simulink model "TSR_EuroNCAP_MSA_ISA_cs"  (R2014b)
settings: Solver=ode5  SolverMode=SingleTasking  StartTime=0.0  StopTime=inf  FixedStep=1/100  RelTol=1e-3
PreLoadFcn:
  | mbxruntime.callbacks.PreLoadFcn(bdroot);
  | check_NUTS_defined;
  | 
  | assignin('base',['model_closed_' bdroot],false);
  | 
  | addpath('../includes_TSR/includes_TSR');
  | 
  | 
  | switch version('-release')
  | case {'2010a', '2010b', '2011a'}
  | addpath('../includes_TSR/ML2010b');
  | otherwise
  | addpath('../includes_TSR/ML2011b');
  | end
PostLoadFcn:
  | mbxruntime.callbacks.PostLoadFcn(bdroot);
InitFcn:
  | mbxruntime.callbacks.InitFcn(bdroot);
StartFcn:
  | mbxruntime.callbacks.StartFcn(bdroot);
StopFcn:
  | mbxruntime.callbacks.StopFcn(bdroot);
model workspace: external: MAT-File .\TSR_EuroNCAP_MSA_ISA_cs_hws.mat (data not in the file)
undefined symbols (not defined in the file or in its folder): InitImageOutputDir, OrientationPitch, OrientationRoll, PositionX, PositionY, PositionZ, warningInitialVelocity, x0
undefined symbols (not defined in the file): SteeringColumn, SteeringWheel, TSR_EuroNCAP_MSA_ISA_cs_0104b7ba9617df32, TSR_EuroNCAP_MSA_ISA_cs_06e8a6c26bfd692b, TSR_EuroNCAP_MSA_ISA_cs_604176ef024b1671, TSR_EuroNCAP_MSA_ISA_cs_9eda5ebf0debb72b, TSR_EuroNCAP_MSA_ISA_cs_aae36e5db6336e11, TSR_EuroNCAP_MSA_ISA_cs_Audi_A8_1_Dynamics_Simple_initialPitch, TSR_EuroNCAP_MSA_ISA_cs_Audi_A8_1_Dynamics_Simple_initialRoll, TSR_EuroNCAP_MSA_ISA_cs_Audi_A8_1_Dynamics_Simple_initialX, TSR_EuroNCAP_MSA_ISA_cs_Audi_A8_1_Dynamics_Simple_initialY, TSR_EuroNCAP_MSA_ISA_cs_Audi_A8_1_Dynamics_Simple_initialYaw, TSR_EuroNCAP_MSA_ISA_cs_Audi_A8_1_Dynamics_Simple_initialZ, TSR_EuroNCAP_MSA_ISA_cs_c75eda1a4a1a144d, TSR_EuroNCAP_MSA_ISA_cs_e3e021b268cede46, WheelL0, WheelL1, WheelR0, WheelR1
libraries: simulink x21, simulink_extras x13, PreScanSimulinkLibrary x5
(part 1 of 6)
CloseFcn:
  | mbxruntime.callbacks.CloseFcn(bdroot);
  | evalin('base',['clear model_closed_' bdroot]);
settings Model: Creator=PRESCAN  LastModifiedBy=jenkins
settings DataIOCC: SignalLoggingSaveFormat=ModelDataLogs
settings OptimizationCC: InlineParams=on  ExpressionDepthLimit=2147483647  InitFltsAndDblsToZero=on
settings DebuggingCC: SaveWithParameterizedLinksMsg=none  UnderspecifiedInitializationDetection=Classic  MergeDetectMultiDrivingBlocksExec=none  SignalResolutionControl=TryResolveAllWithWarning  SolverPrmCheckMsg=none  MultiTaskDSMMsg=warning  MultiTaskCondExecSysMsg=none  FcnCallInpInsideContextMsg=UseLocalSettings  StateNameClashWarn=warning
settings ModelReferenceCC: UpdateModelReferenceTargets=IfOutOfDate
settings SFSimCC: SimParseCustomCode=off
settings SFSimCC: SimCustomHeaderCode=|
  | #include "prescan.h"
  | #include "prescan_platform.h"
settings RTWCC: IncludeERTFirstTime=on
settings GRTTargetCC: TargetFcnLib=ansi_tfl_tmw.mat  CombineOutputUpdateFcns=off  GRTInterface=on

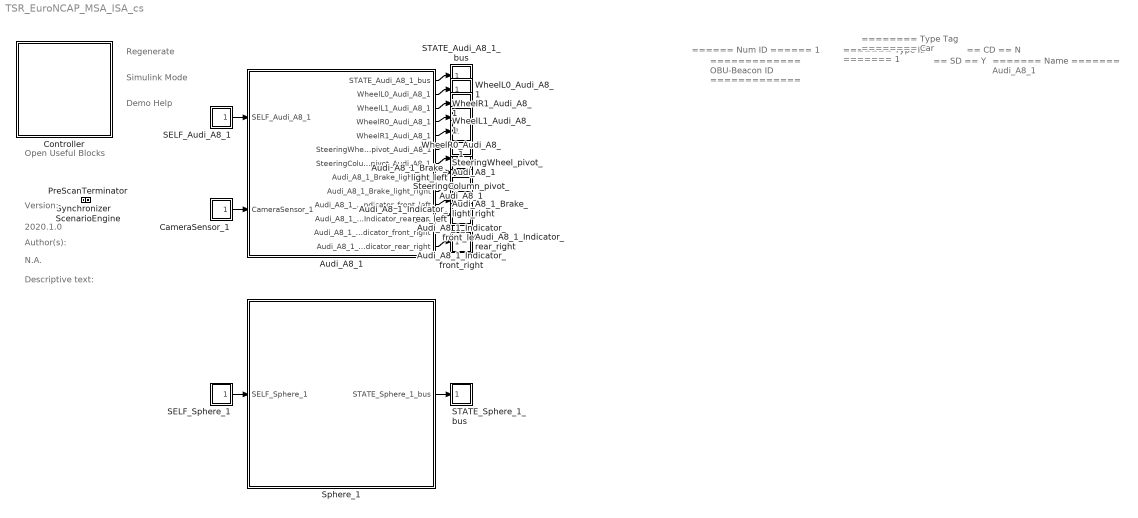
== system TSR_EuroNCAP_MSA_ISA_cs ==
  note: Regenerate
  note: Simulink Mode
  note: Open Useful Blocks
  note: 2020.1.0
  note: Version:
  note: Author(s):
  note: N.A.
  note: Descriptive text:
  note: Demo Help
  note: ======
      | Num ID
      | ======
      | 1
  note: =============
      | OBU-Beacon ID
      | =============
  note: =======
      | Type ID
      | =======
      | 1
  note: ========
      | Type Tag
      | ========
      | Car
  note: ==
      | SD
      | ==
      | Y
  note: ==
      | CD
      | ==
      | N
  note: =======
      | Name
      | =======
      | Audi_A8_1
  Audi_A8_1 : Subsystem  Tag=WorldObjectSubSystem  InitFcn=UniqueId = '253';
      mask init:
      | modelPath = GenericModelHelper.getGenericModelFilePath('ModelDepo','Vehicles\Audi_A8\Audi_A8.pgmb','e33fe1ddcf3e8ae97caccbc8f2fa74ac');imagePath = GenericModelHelper.getCompilationPicture(modelPath, 'Audi_A8_HighPoly.png');
      mask Display: image(imread(imagePath));color('white');text(0, 0, ' ID=1\n')
  Audi_A8_1_Brake_light_left : Subsystem  Tag=actuator/BrakeLightL  Priority=0  LoadFcn=load('PreScanVisuLightActuatorData');load('PrescanRPYData');load('PrescanXYZData');load('PreScanRGBData')  mask(PreScan Sink Block: VisuActiveLight){}
      mask help:
      | The VisuActiveLight block provides a way for detailed animation of Light Sources, such as the indicator, brake, fog and main lights of a vehicle, or a light post.
      |
      | For more information, please click Help.
      settings: OpenFcn=open_system([gcb '/Actuator'],'mask')
      mask Help: eval('openHelp(209)')
      mask Display: image(imread('HeadLight.png'))
  Audi_A8_1_Brake_light_right : Subsystem  Tag=actuator/BrakeLightR  Priority=0  LoadFcn=load('PreScanVisuLightActuatorData');load('PrescanRPYData');load('PrescanXYZData');load('PreScanRGBData')  mask(PreScan Sink Block: VisuActiveLight){}
      mask help:
      | The VisuActiveLight block provides a way for detailed animation of Light Sources, such as the indicator, brake, fog and main lights of a vehicle, or a light post.
      |
      | For more information, please click Help.
      settings: OpenFcn=open_system([gcb '/Actuator'],'mask')
      mask Help: eval('openHelp(209)')
      mask Display: image(imread('HeadLight.png'))
  Audi_A8_1_Indicator_front_left : Subsystem  Tag=actuator/IndicatorFL  Priority=0  LoadFcn=load('PreScanVisuLightActuatorData');load('PrescanRPYData');load('PrescanXYZData');load('PreScanRGBData')  mask(PreScan Sink Block: VisuActiveLight){}
      mask help:
      | The VisuActiveLight block provides a way for detailed animation of Light Sources, such as the indicator, brake, fog and main lights of a vehicle, or a light post.
      |
      | For more information, please click Help.
      settings: OpenFcn=open_system([gcb '/Actuator'],'mask')
      mask Help: eval('openHelp(209)')
      mask Display: image(imread('HeadLight.png'))
  Audi_A8_1_Indicator_front_right : Subsystem  Tag=actuator/IndicatorFR  Priority=0  LoadFcn=load('PreScanVisuLightActuatorData');load('PrescanRPYData');load('PrescanXYZData');load('PreScanRGBData')  mask(PreScan Sink Block: VisuActiveLight){}
      mask help:
      | The VisuActiveLight block provides a way for detailed animation of Light Sources, such as the indicator, brake, fog and main lights of a vehicle, or a light post.
      |
      | For more information, please click Help.
      settings: OpenFcn=open_system([gcb '/Actuator'],'mask')
      mask Help: eval('openHelp(209)')
      mask Display: image(imread('HeadLight.png'))
  Audi_A8_1_Indicator_rear_left : Subsystem  Tag=actuator/IndicatorRL  Priority=0  LoadFcn=load('PreScanVisuLightActuatorData');load('PrescanRPYData');load('PrescanXYZData');load('PreScanRGBData')  mask(PreScan Sink Block: VisuActiveLight){}
      mask help:
      | The VisuActiveLight block provides a way for detailed animation of Light Sources, such as the indicator, brake, fog and main lights of a vehicle, or a light post.
      |
      | For more information, please click Help.
      settings: OpenFcn=open_system([gcb '/Actuator'],'mask')
      mask Help: eval('openHelp(209)')
      mask Display: image(imread('HeadLight.png'))
  Audi_A8_1_Indicator_rear_right : Subsystem  Tag=actuator/IndicatorRR  Priority=0  LoadFcn=load('PreScanVisuLightActuatorData');load('PrescanRPYData');load('PrescanXYZData');load('PreScanRGBData')  mask(PreScan Sink Block: VisuActiveLight){}
      mask help:
      | The VisuActiveLight block provides a way for detailed animation of Light Sources, such as the indicator, brake, fog and main lights of a vehicle, or a light post.
      |
      | For more information, please click Help.
      settings: OpenFcn=open_system([gcb '/Actuator'],'mask')
      mask Help: eval('openHelp(209)')
      mask Display: image(imread('HeadLight.png'))
  CameraSensor_1 : Subsystem  Tag=sensor/Camera/CameraSensor  Priority=30  mask(PreScan Source Block: Camera Sensor){}
      mask help: The Camera Sensor provides a color or monochrome image.
      settings: OpenFcn=open_system([gcb '/Sensor'],'mask')
      mask Help: eval('openHelp(457)')
      mask Display: image(imread('CameraSensor.png'))
  Controller : Subsystem  Description=8A3CD2955739A82C886C20AE3E253D78460D53180EE2C1B14CC08DF75A70BE77  Priority=-1  LoadFcn=load PreScanControllerData  mask(PreScan Simulation Controller){prescanversion='2020.1.0', ModelReferencing=off, TimeStep=1/100, ControlMode=0, PreScanExecutionMode=on, ControllerCount=0, ControllerIndex=0, ControllerOptions=''}
      mask prompts: prescanversion "PreScan Version"; ModelReferencing "Use Model Referencing"; TimeStep "Upload Period [s]"; ControlMode "Control Mode"; PreScanExecutionMode "Execution Mode"; ControllerCount "Controller Count"; ControllerIndex "Controller Index"; ControllerOptions "Controller Options"
      mask help:
      | Please do not remove this block from the compilation sheet,
      | as it connects the model to the PreScan environment.
      mask init:
      | model = bdroot(gcb);
      | ExperimentFile = mbxruntime.findExperimentFile(model,true); %relative path
      | 
      | [d1, d2, d3, prescandata] = prescan_Settings();
      | ModelDepo = fullfile(prescandata,'ModelDepo'); 
      | 
      | RTmode = mbxruntime.getRTMode(model);
      | 
      | SimulationMode = get_param(bdroot,'SimulationMode');
      | if strcmp(SimulationMode, 'rapid-accelerator')
      |     SimulationMode = 'external';
      | end
      | TargetName = get_param(bdroot,'SystemTargetFile');
      settings: ModelCloseFcn=assignin('base',['model_closed_' bdroot],true);
      mask Help: eval('openHelp(812)')
      mask Display: image(imread('prescanlogo.ico'))
  PreScanTerminator : Subsystem  Tag=PreScanTerminator  Priority=999  LoadFcn=load PrescanTerminatorData  mask(PreScan Simulation Terminator){TimeStep=1/100}
      mask prompts: TimeStep "Upload Period [s]"
      mask help:
      | Please do not remove this block from the compilation sheet as it
      | connects the model to the PreScan environment.
      mask Help: eval('openHelp(812)')
      mask Display: image(imread('prescanlogo.ico'))
  SELF_Audi_A8_1 : Subsystem  Tag=sensor/SelfPort  Priority=30  LoadFcn=load('PreScanSelfSensorData.mat')  mask(PreScan Source Block: SELF){}
      mask help:
      | The SELF port shows (state) information of the actor itself. The outputs are position in the experiment's axis system and the GPS coordinates, and the object's absolute velocity and compass heading.
      |
      | For more information, please click Help.
      settings: OpenFcn=open_system([gcb '/Sensor'],'mask')
      mask Help: eval('openHelp(462)')
      mask Display: image(imread('GPS.png'))
  SELF_Sphere_1 : Subsystem  Tag=sensor/SelfPort  Priority=30  LoadFcn=load('PreScanSelfSensorData.mat')  mask(PreScan Source Block: SELF){}
      mask help:
      | The SELF port shows (state) information of the actor itself. The outputs are position in the experiment's axis system and the GPS coordinates, and the object's absolute velocity and compass heading.
      |
      | For more information, please click Help.
      settings: OpenFcn=open_system([gcb '/Sensor'],'mask')
      mask Help: eval('openHelp(462)')
      mask Display: image(imread('GPS.png'))
  STATE_Audi_A8_1_bus : Subsystem  Tag=actuator/StatePort  Priority=0  LoadFcn=load('PreScanStateActuatorData.mat')  mask(PreScan Sink Block: State){}
      mask help:
      | The Actor State contains a vector signal of size (9x1), containing the following signals:
      |
      | -  Position    	(x,y,z)             	[m]
      | -  Velocity    	(vx,vy,vz)         	[m/s]
      | -  Angles       	(Roll, Pitch, Yaw)	[rad]
      |
      | The Actor state is defined in the global axis system.
      | The state is superponed on the Initial position defined in the GUI.
      |
      | For more information, please click Help.
      settings: OpenFcn=open_system([gcb '/Actuator'],'mask')
      mask Help: eval('openHelp(222)')
      mask Display: image(imread('State.png'))
  STATE_Sphere_1_bus : Subsystem  Tag=actuator/StatePort  Priority=0  LoadFcn=load('PreScanStateActuatorData.mat')  mask(PreScan Sink Block: State){}
      mask help:
      | The Actor State contains a vector signal of size (9x1), containing the following signals:
      |
      | -  Position    	(x,y,z)             	[m]
      | -  Velocity    	(vx,vy,vz)         	[m/s]
      | -  Angles       	(Roll, Pitch, Yaw)	[rad]
      |
      | The Actor state is defined in the global axis system.
      | The state is superponed on the Initial position defined in the GUI.
      |
      | For more information, please click Help.
      settings: OpenFcn=open_system([gcb '/Actuator'],'mask')
      mask Help: eval('openHelp(222)')
      mask Display: image(imread('State.png'))
  ScenarioEngine : Subsystem  Tag=PreScanOpenScenarioBlock  Priority=10  LoadFcn=load PrescanSynchronizeData  mask(PreScan Simulation Core Block){TimeStep=1/100}
      mask prompts: TimeStep "Timestep [s]"
      mask help:
      | Please do not remove this block from the PreScan compilation sheet,
      | as it contains essential configuration parameters for a PreScan simulation.
      settings: DeleteFcn=PreScanBlockDeleteFcn;
      mask Display: image(imread('prescanlogo.ico'))
  Sphere_1 : Subsystem  Tag=WorldObjectSubSystem  InitFcn=UniqueId = '277';
      mask init:
      | imagePath=which('Sphere.jpg');
      mask Display: image(imread(imagePath));color('white');text(0, 0, ' ID=2\n')
  SteeringColumn_pivot_Audi_A8_1 : Subsystem  Tag=Actuator  Priority=0  LoadFcn=load('PrescanPoseData');load('PrescanXYZData');load('PreScanRPYData')
      mask help:
      | The VisuJoint block provides a way to adapt the location and orientation of a part of an object.
      |
      | For more information, please click Help.
      settings: OpenFcn=open_system([gcb '/Actuator'],'mask')
      mask Display: image(imread('Joint.png'))
  SteeringWheel_pivot_Audi_A8_1 : Subsystem  Tag=Actuator  Priority=0  LoadFcn=load('PrescanPoseData');load('PrescanXYZData');load('PreScanRPYData')
      mask help:
      | The VisuJoint block provides a way to adapt the location and orientation of a part of an object.
      |
      | For more information, please click Help.
      settings: OpenFcn=open_system([gcb '/Actuator'],'mask')
      mask Display: image(imread('Joint.png'))
  Synchronizer : Subsystem  Tag=PreScanSynchronizer  Priority=20  LoadFcn=load PrescanSynchronizeData  mask(PreScan Simulation Core Block){TimeStep=1/100}
      mask prompts: TimeStep "Timestep [s]"
      mask help:
      | Please do not remove this block from the PreScan compilation sheet,
      | as it contains essential configuration parameters for a PreScan simulation.
      settings: DeleteFcn=PreScanBlockDeleteFcn;
      mask Display: image(imread('prescanlogo.ico'))
  WheelL0_Audi_A8_1 : Subsystem  Tag=Actuator  Priority=0  LoadFcn=load('PrescanPoseData');load('PrescanXYZData');load('PreScanRPYData')
      mask help:
      | The VisuJoint block provides a way to adapt the location and orientation of a part of an object.
      |
      | For more information, please click Help.
      settings: OpenFcn=open_system([gcb '/Actuator'],'mask')
      mask Display: image(imread('Joint.png'))
  WheelL1_Audi_A8_1 : Subsystem  Tag=Actuator  Priority=0  LoadFcn=load('PrescanPoseData');load('PrescanXYZData');load('PreScanRPYData')
      mask help:
      | The VisuJoint block provides a way to adapt the location and orientation of a part of an object.
      |
      | For more information, please click Help.
      settings: OpenFcn=open_system([gcb '/Actuator'],'mask')
      mask Display: image(imread('Joint.png'))
  WheelR0_Audi_A8_1 : Subsystem  Tag=Actuator  Priority=0  LoadFcn=load('PrescanPoseData');load('PrescanXYZData');load('PreScanRPYData')
      mask help:
      | The VisuJoint block provides a way to adapt the location and orientation of a part of an object.
      |
      | For more information, please click Help.
      settings: OpenFcn=open_system([gcb '/Actuator'],'mask')
      mask Display: image(imread('Joint.png'))
  WheelR1_Audi_A8_1 : Subsystem  Tag=Actuator  Priority=0  LoadFcn=load('PrescanPoseData');load('PrescanXYZData');load('PreScanRPYData')
      mask help:
      | The VisuJoint block provides a way to adapt the location and orientation of a part of an object.
      |
      | For more information, please click Help.
      settings: OpenFcn=open_system([gcb '/Actuator'],'mask')
      mask Display: image(imread('Joint.png'))
  wires:
  Audi_A8_1/1(STATE_Audi_A8_1_bus) -> STATE_Audi_A8_1_bus/1(STATE_Audi_A8_1_bus)
  SELF_Audi_A8_1/1(SELF_Audi_A8_1) -> Audi_A8_1/1(SELF_Audi_A8_1)
  CameraSensor_1/1(CameraSensor_1) -> Audi_A8_1/2(CameraSensor_1)
  Audi_A8_1/2(WheelL0_Audi_A8_1) -> WheelL0_Audi_A8_1/1(WheelL0_Audi_A8_1)
  Audi_A8_1/3(WheelL1_Audi_A8_1) -> WheelL1_Audi_A8_1/1(WheelL1_Audi_A8_1)
  Audi_A8_1/4(WheelR0_Audi_A8_1) -> WheelR0_Audi_A8_1/1(WheelR0_Audi_A8_1)
  Audi_A8_1/5(WheelR1_Audi_A8_1) -> WheelR1_Audi_A8_1/1(WheelR1_Audi_A8_1)
  Audi_A8_1/6(SteeringWheel_pivot_Audi_A8_1) -> SteeringWheel_pivot_Audi_A8_1/1(SteeringWheel_pivot_Audi_A8_1)
  Audi_A8_1/7(SteeringColumn_pivot_Audi_A8_1) -> SteeringColumn_pivot_Audi_A8_1/1(SteeringColumn_pivot_Audi_A8_1)
  Audi_A8_1/8(Audi_A8_1_Brake_light_left) -> Audi_A8_1_Brake_light_left/1(Audi_A8_1_Brake_light_left)
  Audi_A8_1/9(Audi_A8_1_Brake_light_right) -> Audi_A8_1_Brake_light_right/1(Audi_A8_1_Brake_light_right)
  Audi_A8_1/10(Audi_A8_1_Indicator_front_left) -> Audi_A8_1_Indicator_front_left/1(Audi_A8_1_Indicator_front_left)
  Audi_A8_1/11(Audi_A8_1_Indicator_rear_left) -> Audi_A8_1_Indicator_rear_left/1(Audi_A8_1_Indicator_rear_left)
  Audi_A8_1/12(Audi_A8_1_Indicator_front_right) -> Audi_A8_1_Indicator_front_right/1(Audi_A8_1_Indicator_front_right)
  Audi_A8_1/13(Audi_A8_1_Indicator_rear_right) -> Audi_A8_1_Indicator_rear_right/1(Audi_A8_1_Indicator_rear_right)
  Sphere_1/1(STATE_Sphere_1_bus) -> STATE_Sphere_1_bus/1(STATE_Sphere_1_bus)
  SELF_Sphere_1/1(SELF_Sphere_1) -> Sphere_1/1(SELF_Sphere_1)

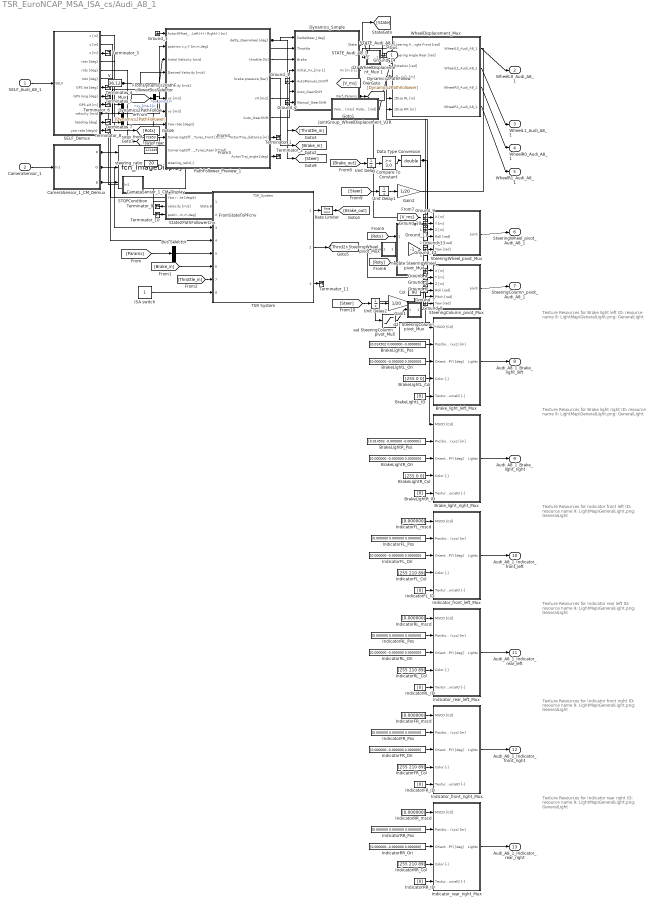
== system TSR_EuroNCAP_MSA_ISA_cs/Audi_A8_1 ==
  note: Texture Resources for Brake light left
      |
      | ID: resource name
      | 9: LightMap\GeneralLight.png: GeneralLight
  note: Texture Resources for Brake light right
      |
      | ID: resource name
      | 9: LightMap\GeneralLight.png: GeneralLight
  note: Texture Resources for Indicator front left
      |
      | ID: resource name
      | 9: LightMap\GeneralLight.png: GeneralLight
  note: Texture Resources for Indicator rear left
      |
      | ID: resource name
      | 9: LightMap\GeneralLight.png: GeneralLight
  note: Texture Resources for Indicator front right
      |
      | ID: resource name
      | 9: LightMap\GeneralLight.png: GeneralLight
  note: Texture Resources for Indicator rear right
      |
      | ID: resource name
      | 9: LightMap\GeneralLight.png: GeneralLight
  SELF_Audi_A8_1 : Inport  Tag=inport/SelfPort  OutDataTypeStr=Bus: PRESCAN_SELFSENSORDATA  PortDimensions=1  SampleTime=1/100  BusOutputAsStruct=on
  CameraSensor_1 : Inport  Tag=inport/Camera/CameraSensor  Port=2  OutDataTypeStr=uint8  SampleTime=1/50  BusOutputAsStruct=on
  " " : Subsystem  mask{da=1.17, db=1.77, h=0.21, w=1.612}
      mask prompts: da "Distance to the front wheel from cars center of gravity [m]"; db "Distance to the back wheel from cars center of gravity [m]"; h "Center of gravity height [m]"; w "Width of the car [m]"
      mask init:
      | a  = sqrt( da*da + h*h );
      | b  = sqrt( db*db + h*h );
      | TW = sqrt( 0.25*w*w + h*h );
  BrakeLightL_Col : Constant  Tag=VisuLightConst  Value=[255 0 0]
  BrakeLightL_ID : Constant  Tag=VisuLightConst  Value=[0]
  BrakeLightL_Ori : Constant  Tag=VisuLightConst  Value=[0.000000 -0.000000 0.000000]
  BrakeLightL_Pos : Constant  Tag=VisuLightConst  Value=[0.014502 0.000000 -0.000000]
  BrakeLightR_Col : Constant  Tag=VisuLightConst  Value=[255 0 0]
  BrakeLightR_ID : Constant  Tag=VisuLightConst  Value=[0]
  BrakeLightR_Ori : Constant  Tag=VisuLightConst  Value=[0.000000 -0.000000 0.000000]
  BrakeLightR_Pos : Constant  Tag=VisuLightConst  Value=[0.014502 -0.000000 -0.000000]
  Brake_light_left_Mux : Subsystem  Tag=mux/ActiveLight  mask(PreScan User Interface: VisuActiveLight){}
      mask help:
      | The VisuActiveLight block provides a way for detailed animation of Light Sources, such as the indicator, brake, fog and main lights of a vehicle, or a light post.
      |
      | For more information, please click Help.
      settings: DeleteFcn=PreScanBlockDeleteFcn;
      mask Help: eval('openHelp(209)')
  Brake_light_right_Mux : Subsystem  Tag=mux/ActiveLight  mask(PreScan User Interface: VisuActiveLight){}
      mask help:
      | The VisuActiveLight block provides a way for detailed animation of Light Sources, such as the indicator, brake, fog and main lights of a vehicle, or a light post.
      |
      | For more information, please click Help.
      settings: DeleteFcn=PreScanBlockDeleteFcn;
      mask Help: eval('openHelp(209)')
  Bus Selector : BusSelector  OutputSignals=NEngine_[rpm]
  CameraSensor_1_CM_Demux : Subsystem  Tag=demux/Camera/Color  mask{SensorName=CameraSensor_1, hres=800, vres=600}
      mask prompts: SensorName "Sensor Name"; hres "Horizontal Resolution"; vres "Vertical Resolution"
      mask Help: eval('openHelp(457)')
      mask Display:
      | fprintf('MONO CAMERA:\n Color\n %s \n %d x %d px',SensorName,hres,vres)
      | port_label('output',1,'R')
      | port_label('output',2,'G')
      | port_label('output',3,'B')
  CameraSensor_1_CM_Display : M-S-Function  Tag=CameraSensor_Color_Display  InitFcn=InitImageOutputDir(gcb);  FunctionName=fcn_ImageDisplay  Parameters=SensorName EnableDisplay EnablePosition DisplayPosition FigureHandle SaveResults BitmapFormat TempOutputDir CameraType DataType  mask(PreScan Color Display Block){SensorName=CameraSensor_1, EnableDisplay=on, EnablePosition=off, DisplayPosition=[10 10 800 600], FigureHandle=25301, SaveResults=off, Format=PNG, TempOutputDir=0, CameraType=Mono, DataType=uint8}
      mask prompts: SensorName "User Specified: Title of Display"; EnableDisplay "Active"; EnablePosition "Set Display window position"; DisplayPosition "Display window position [xpos ypos width height]"; FigureHandle "Unique Handle"; SaveResults "Save results"; TempOutputDir "OutputDir"; CameraType "Camera Type"; DataType "Image Data Type"
      mask help: This block displays the RGB output of a PreScan camera sensor.
      mask init:
      | if EnableDisplay
      |     EnableString='';
      |     EnableColor='gray';
      | else
      |     EnableString='INACTIVE';
      |     EnableColor='red';
      | end
      | switch Format
      |     case 1
      |         BitmapFormat = 'png';
      |     case 2
      |         BitmapFormat = 'bmp';
      |     case 3
      |         BitmapFormat = 'jpg';
      | end 
      | if CameraType==1
      |     CameraTypeName='MONO';
      |     PortNumber=0;
      | else
      |     CameraTypeName='STEREO';
      |     PortNumber=3;
      | end
      settings: CopyFcn=CopyFcnDisplay  DeleteFcn=PreScanBlockDeleteFcn;  ModelCloseFcn=fcn_ImageDisplay_ModelCloseFcn
      mask Help: eval('openHelp(457)')
      mask Callback EnablePosition:
      | MV=get_param(gcb,'MaskVisibilities');
      | if strcmp(get_param(gcb,'EnablePosition'),'on')
      |     MV{4}='on';
      | else
      |     MV{4}='off';
      | end
      | set_param(gcb,'MaskVisibilities',MV);
      | clear MV;
      mask TypeOptions Format: PNG | BMP | JPG
      mask TypeOptions CameraType: Mono | Stereo
      mask TypeOptions DataType: uint8 | single
      mask Display:
      | color(EnableColor);
      | fprintf('%s\n DISPLAY:\n Color \n %s',EnableString,SensorName)
      | port_label('input',1,'R')
      | port_label('input',2,'G')
      | port_label('input',3,'B')
      | port_label('input',PortNumber+1,'R')
      | port_label('input',PortNumber+2,'G')
      | port_label('input',PortNumber+3,'B')
  Col : Constant  Value=90
  Compare To Constant : simulink/Logic and Bit Operations/Compare To Constant  relop=>=  const=3.0  OutDataTypeStr=boolean
  Data Type Conversion : DataTypeConversion  OutDataTypeStr=double
  Dynamics_Simple : Subsystem  Tag=Simple_Vehicle_Dynamics  mask(PreScan Block: Simple Dynamics){TimeStep=1/100, ComputationMode=Continuous_Time, initialX=TSR_EuroNCAP_MSA_ISA_cs_Audi_A8_1_Dynamics_Simple_initialX, initialY=TSR_EuroNCAP_MSA_ISA_cs_Audi_A8_1_Dynamics_Simple_initialY, initialZ=TSR_EuroNCAP_MSA_ISA_cs_Audi_A8_1_Dynamics_Simple_initialZ, initialRoll=TSR_EuroNCAP_MSA_ISA_cs_Audi_A8_1_Dynamics_Simple_initialRoll, initialPitch=TSR_EuroNCAP_MSA_ISA_cs_Audi_A8_1_Dynamics_Simple_initialPitch, initialYaw=TSR_EuroNCAP_MSA_ISA_cs_Audi_A8_1_Dynamics_Simple_initialYaw}
      mask prompts: TimeStep "Auto assigned: Time Step [s]"; ComputationMode "Computation mode:"; initialX "Ini x-position VEHICLE wrt GLOBAL axis system [m]"; initialY "Ini y-position VEHICLE wrt GLOBAL axis system [m]"; initialZ "Ini z-position VEHICLE wrt GLOBAL axis system [m]"; initialRoll "Ini roll-angle BODY wrt VEHICLE axis system [deg]"; initialPitch "Ini pitch-angle BODY wrt VEHICLE axis system [deg]"; initialYaw "Ini yaw-angle VEHICLE wrt GLOBAL axis system [deg]"
      mask help:
      | The Simple Dynamics Model is selected in the GUI to simulate vehicle dynamics behavior.
      |
      | The Simple Dynamics Model is completely open to the user. The parameters of this model can be set in the Simple Dynamics dialog in the GUI.
      |
      | For more information, please click Help.
      mask init:
      | p = SimpleDyn_pars;
      settings: DeleteFcn=PreScanBlockDeleteFcn;
      mask Help: eval('openHelp(220)')
      mask Display:
      | image(imread('SimpleDyn.png'))
      | port_label('input', 1, '{\delta}_S_t_ _e_e_r [deg]','texmode','on')
      | port_label('input', 2, 'Throttle [%]')
      | port_label('input', 3, 'Brake Pres [bar]')
      | port_label('input', 4, 'V_0 [ms-1]','texmode','on')
      | port_label('input', 5, 'Auto=[0]/Manual=[1]')
      | port_label('input', 6, 'Auto_GearShift')
      | port_label('input', 7, 'Manual_GearShift')
      | port_label('output', 1, 'State')
      | port_label('output', 2, 'Vx [ms-1]')
      | port_label('output', 3, 'Perf Params')
  FromDynamics2PathFollowerBusSelector : BusSelector  OutputSignals=vx_[ms-1],vy_[ms-1]
  Gain1 : Gain  Gain=1/20
  Gain2 : Gain  Gain=1/20
  Ground_{1..14} (14 alike) : Ground
  ISA switch : Constant
  IndicatorFL_Col : Constant  Tag=VisuLightConst  Value=[255 210 89]
  IndicatorFL_ID : Constant  Tag=VisuLightConst  Value=[0]
  IndicatorFL_Ori : Constant  Tag=VisuLightConst  Value=[0.000000 -0.000000 0.000000]
  IndicatorFL_Pos : Constant  Tag=VisuLightConst  Value=[0.000000 0.000000 0.000000]
  IndicatorFL_mscd : Constant  Tag=VisuLightConst  Value=[0.000000]
  IndicatorFR_Col : Constant  Tag=VisuLightConst  Value=[255 210 89]
  IndicatorFR_ID : Constant  Tag=VisuLightConst  Value=[0]
  IndicatorFR_Ori : Constant  Tag=VisuLightConst  Value=[0.000000 -0.000000 0.000000]
  IndicatorFR_Pos : Constant  Tag=VisuLightConst  Value=[0.000000 0.000000 0.000000]
  IndicatorFR_mscd : Constant  Tag=VisuLightConst  Value=[0.000000]
  IndicatorRL_Col : Constant  Tag=VisuLightConst  Value=[255 210 89]
  IndicatorRL_ID : Constant  Tag=VisuLightConst  Value=[0]
  IndicatorRL_Ori : Constant  Tag=VisuLightConst  Value=[0.000000 -0.000000 0.000000]
  IndicatorRL_Pos : Constant  Tag=VisuLightConst  Value=[0.000000 0.000000 0.000000]
  IndicatorRL_mscd : Constant  Tag=VisuLightConst  Value=[0.000000]
  IndicatorRR_Col : Constant  Tag=VisuLightConst  Value=[255 210 89]
  IndicatorRR_ID : Constant  Tag=VisuLightConst  Value=[0]
  IndicatorRR_Ori : Constant  Tag=VisuLightConst  Value=[0.000000 -0.000000 0.000000]
  IndicatorRR_Pos : Constant  Tag=VisuLightConst  Value=[0.000000 0.000000 0.000000]
  IndicatorRR_mscd : Constant  Tag=VisuLightConst  Value=[0.000000]
  Indicator_front_left_Mux : Subsystem  Tag=mux/ActiveLight  mask(PreScan User Interface: VisuActiveLight){}
      mask help:
      | The VisuActiveLight block provides a way for detailed animation of Light Sources, such as the indicator, brake, fog and main lights of a vehicle, or a light post.
      |
      | For more information, please click Help.
      settings: DeleteFcn=PreScanBlockDeleteFcn;
      mask Help: eval('openHelp(209)')
  Indicator_front_right_Mux : Subsystem  Tag=mux/ActiveLight  mask(PreScan User Interface: VisuActiveLight){}
      mask help:
      | The VisuActiveLight block provides a way for detailed animation of Light Sources, such as the indicator, brake, fog and main lights of a vehicle, or a light post.
      |
      | For more information, please click Help.
      settings: DeleteFcn=PreScanBlockDeleteFcn;
      mask Help: eval('openHelp(209)')
  Indicator_rear_left_Mux : Subsystem  Tag=mux/ActiveLight  mask(PreScan User Interface: VisuActiveLight){}
      mask help:
      | The VisuActiveLight block provides a way for detailed animation of Light Sources, such as the indicator, brake, fog and main lights of a vehicle, or a light post.
      |
      | For more information, please click Help.
      settings: DeleteFcn=PreScanBlockDeleteFcn;
      mask Help: eval('openHelp(209)')
  Indicator_rear_right_Mux : Subsystem  Tag=mux/ActiveLight  mask(PreScan User Interface: VisuActiveLight){}
      mask help:
      | The VisuActiveLight block provides a way for detailed animation of Light Sources, such as the indicator, brake, fog and main lights of a vehicle, or a light post.
      |
      | For more information, please click Help.
      settings: DeleteFcn=PreScanBlockDeleteFcn;
      mask Help: eval('openHelp(209)')
  JointGroup_WheelDisplacement_V2R : Subsystem  Tag=mux/Wheels  mask(PreScan Velocity to Wheel Angle Block:){TimeStep=1/100, TireRadius=0.34}
      mask prompts: TimeStep "Auto Assigned: Time Step [s]"; TireRadius "Tire Radius [m]"
      settings: DeleteFcn=PreScanBlockDeleteFcn;
      mask Display: disp('Velocity\nto\nWheelAngle')
  Mux : Mux  Inputs=3
  PathFollower_Preview_1 : Subsystem  Tag=PathFollower_Preview  mask(PreScan Block: Path Follower with Preview){LongCtrl_P=20, LongCtrl_I=0.3, LongCtrl_D=3.065, LongCtrl_AWU=1, LongCtrlDefault_P=20, LongCtrlDefault_I=0.3, LongCtrlDefault_D=3.065, LongCtrlDefault_AWU=1, PathUniqueID=TSR_EuroNCAP_MSA_ISA_cs_c75eda1a4a1a144d, mass=1820, Jzz=3746, length_a=1.17, length_l=2.94, Angle_Max_SteeringWheel=500, PreviewTime=1, DelayTime=0.1, LowSpeedLimit=20, MaxSteeringRate=1200, CSSampleTime=1/100, PFIntegrationFrequency=100}
      mask prompts: LongCtrl_P "Longitudinal Controller P"; LongCtrl_I "Longitudinal Controller I"; LongCtrl_D "Longitudinal Controller D"; LongCtrl_AWU "Longitudinal Controller AWU"; PathUniqueID "Path Unique ID"; mass "Mass vehicle total [kg]"; Jzz "Inertia vehicle around yaw axis [kg m2]"; length_a "Distance between COG and front axle [m]"; length_l "Length of wheelbase [m]"; Angle_Max_SteeringWheel "Maximum steering wheel angle [deg]"; PreviewTime "Preview time [s]"; DelayTime "Delay time [s]"; LowSpeedLimit "Low-speed limit [km/h]"; MaxSteeringRate "Maximum steering wheel angle rate [deg/s]"; CSSampleTime "Compilation Sheet sample time [s]"; PFIntegrationFrequency "Lateral controller frequency [Hz]"
      mask help:
      | The Path Follower Model is selected in the GUI to simulate driver behavior.
      |
      | For more information, please click Help.
      mask init:
      | RefreshCounter = max(floor((1/CSSampleTime) / (PFIntegrationFrequency)), 1);
      | PathFollowerBlockPath = gcb;
      mask Help: eval('openHelp(233)')
      mask DialogControl Control2 Prompt: Reset PID parameters
      mask DialogControl Control2 Callback:
      | LongCtrlDefault_P = get_param(gcb,'LongCtrlDefault_P');
      | set_param(gcb,'LongCtrl_P',LongCtrlDefault_P);
      | 
      | LongCtrlDefault_I = get_param(gcb,'LongCtrlDefault_I');
      | set_param(gcb,'LongCtrl_I',LongCtrlDefault_I);
      | 
      | LongCtrlDefault_D = get_param(gcb,'LongCtrlDefault_D');
      | set_param(gcb,'LongCtrl_D',LongCtrlDefault_D);
      | 
      | LongCtrlDefault_AWU = get_param(gcb,'LongCtrlDefault_AWU');
      | set_param(gcb,'LongCtrl_AWU',LongCtrlDefault_AWU);
  Rate Limiter : RateLimiter  RisingSlewLimit=150  FallingSlewLimit=-150  SampleTimeMode=inherited
  SELF_Demux : Subsystem  Tag=demux/SelfPort  mask(PreScan Demux Block:){}
      mask help:
      | The SELF port shows (state) information of the actor itself. The outputs are position in the experiment's axis system and the GPS coordinates, and the object's absolute velocity and compass heading.
      |
      | For more information, please click Help.
      settings: DeleteFcn=PreScanBlockDeleteFcn;
      mask Help: eval('openHelp(462)')
      mask Display:
      | port_label('output',1,'x [m]')
      | port_label('output',2,'y [m]')
      | port_label('output',3,'z [m]','texmode','on')
      | port_label('output',4,'Rotx [deg]','texmode','on')
      | port_label('output',5,'Roty [deg]','texmode','on')
      | port_label('output',6,'Rotz [deg]','texmode','on')
      | port_label('output',7,'GPS lat [deg]','texmode','on')
      | port_label('output',8,'GPS long [deg]','texmode','on')
      | port_label('output',9,'GPS alt [m]','texmode','on')
      | port_label('output',10,'Velocity [m/s]')
      | port_label('output',11,'Heading [deg]')
      | port_label('output',12,'Yaw rate [deg/s]')
  STATE_Audi_A8_1_rc : RateTransition  Tag=mux_rc/StatePort  OutPortSampleTimeOpt=Inherit
  STOPCondition : Subsystem
  State2PathFollowerCnv : Subsystem  Tag=State2PFConnection/cnv
  SteeringColumn_pivot_Mux : Subsystem  Tag=mux/Joint  mask(PreScan Mux Block){DisplayName=SteeringColumn}
      mask prompts: DisplayName "Display Name"
      mask help:
      | This block simulates a generic joint used for generic models. This joint can be enabled/disabled from the GUI.
      |
      | For more information, please click Help.
      settings: DeleteFcn=PreScanBlockDeleteFcn;
      mask Help: eval('openHelp(254)')
  SteeringWheel_pivot_Mux : Subsystem  Tag=mux/Joint  mask(PreScan Mux Block){DisplayName=SteeringWheel}
      mask prompts: DisplayName "Display Name"
      mask help:
      | This block simulates a generic joint used for generic models. This joint can be enabled/disabled from the GUI.
      |
      | For more information, please click Help.
      settings: DeleteFcn=PreScanBlockDeleteFcn;
      mask Help: eval('openHelp(254)')
  TSR System : ModelReference  ModelNameDialog=TSR_System  SimulationMode=Normal  ModelReferenceVersion=1.1003  CopyOfModelName=TSR_System  DefaultDataLogging=off
  Terminator_{1..11} (11 alike) : Terminator
  Unit Delay : UnitDelay  SampleTime=-1
  Unit Delay1 : UnitDelay  SampleTime=-1
  Unit Delay2 : UnitDelay  SampleTime=-1
  V : Constant  Value=36.12
  WheelDisplacement_Mux : Subsystem  Tag=mux/JointGroup  mask(JointGroup){}
      mask help:
      | The JointGroup allows to control several Joints in one go, as defined for this particular model.
      | For more information, look in the PreScan manual in the section "Model Preparation Tool" -> "Joint Groups"
      |
      | For more information on the Joints simulink interface, press Help.
      mask Help: eval('openHelp(254)')
  d2r SteeringColumn_pivot_Mux : Subsystem  mask(DegreesToRadians){}
      mask help: SimulinkBlocks:simulink_extras:DegreesToRadians_MD
      mask Help: web([docroot '/simulink/ref_extras/degreestoradians.html'])
      mask Display: disp('D2R')
  d2r SteeringWheel_pivot_Mux : Subsystem  mask(DegreesToRadians){}
      mask help: SimulinkBlocks:simulink_extras:DegreesToRadians_MD
      mask Help: web([docroot '/simulink/ref_extras/degreestoradians.html'])
      mask Display: disp('D2R')
  d2r WheelDisplacement_Mux 1 : Subsystem  mask(DegreesToRadians){}
      mask help: SimulinkBlocks:simulink_extras:DegreesToRadians_MD
      mask Help: web([docroot '/simulink/ref_extras/degreestoradians.html'])
      mask Display: disp('D2R')
  negate SteeringWheel_pivot_Mux : Gain  Gain=-1
  sat SteeringColumn_pivot_Mux : Saturate  UpperLimit=30  LowerLimit=-5
  steering_ratio : Constant  Tag=steering_ratio  Value=20
  susp_front : Constant  Tag=susp_front  Value=72653
  susp_rear : Constant  Tag=susp_rear  Value=121449
  STATE_Audi_A8_1_bus : Outport  Tag=outport/StatePort  OutDataTypeStr=Bus: PRESCAN_STATEACTUATORDATA  PortDimensions=1  SampleTime=1/100
  WheelL0_Audi_A8_1 : Outport  Tag=outport/JointActuator  Port=2  OutDataTypeStr=Bus: PRESCAN_POSE_DATA  SampleTime=1/100
  WheelL1_Audi_A8_1 : Outport  Tag=outport/JointActuator  Port=3  OutDataTypeStr=Bus: PRESCAN_POSE_DATA  SampleTime=1/100
  WheelR0_Audi_A8_1 : Outport  Tag=outport/JointActuator  Port=4  OutDataTypeStr=Bus: PRESCAN_POSE_DATA  SampleTime=1/100
  WheelR1_Audi_A8_1 : Outport  Tag=outport/JointActuator  Port=5  OutDataTypeStr=Bus: PRESCAN_POSE_DATA  SampleTime=1/100
  SteeringWheel_pivot_Audi_A8_1 : Outport  Tag=outport/JointActuator  Port=6  OutDataTypeStr=Bus: PRESCAN_POSE_DATA  SampleTime=1/100
  SteeringColumn_pivot_Audi_A8_1 : Outport  Tag=outport/JointActuator  Port=7  OutDataTypeStr=Bus: PRESCAN_POSE_DATA  SampleTime=1/100
  Audi_A8_1_Brake_light_left : Outport  Tag=outport/BrakeLightL  Port=8  OutDataTypeStr=Bus: PRESCAN_VISULIGHTACTUATOR_DATA  SampleTime=1/100
  Audi_A8_1_Brake_light_right : Outport  Tag=outport/BrakeLightR  Port=9  OutDataTypeStr=Bus: PRESCAN_VISULIGHTACTUATOR_DATA  SampleTime=1/100
  Audi_A8_1_Indicator_front_left : Outport  Tag=outport/IndicatorFL  Port=10  OutDataTypeStr=Bus: PRESCAN_VISULIGHTACTUATOR_DATA  SampleTime=1/100
  Audi_A8_1_Indicator_rear_left : Outport  Tag=outport/IndicatorRL  Port=11  OutDataTypeStr=Bus: PRESCAN_VISULIGHTACTUATOR_DATA  SampleTime=1/100
  Audi_A8_1_Indicator_front_right : Outport  Tag=outport/IndicatorFR  Port=12  OutDataTypeStr=Bus: PRESCAN_VISULIGHTACTUATOR_DATA  SampleTime=1/100
  Audi_A8_1_Indicator_rear_right : Outport  Tag=outport/IndicatorRR  Port=13  OutDataTypeStr=Bus: PRESCAN_VISULIGHTACTUATOR_DATA  SampleTime=1/100
  tag scope: State=global
  wires:
  [Rotx] -> " "/1(rotX [deg])
  [Roty] -> " "/2(rotY [deg])
  " "/1(zDisp FL [m]) -> WheelDisplacement_Mux/4(zDisp FL [m])
  " "/2(zDisp FR [m]) -> WheelDisplacement_Mux/5(zDisp FR [m])
  " "/3(zDisp RL [m]) -> WheelDisplacement_Mux/6(zDisp RL [m])
  " "/4(zDisp RR [m]) -> WheelDisplacement_Mux/7(zDisp RR [m])
  Bus Selector/1 -> TSR System/5
  TSR System/1 -> Rate Limiter/1
  Rate Limiter/1 -> [Brake_out]
  TSR System/2 -> [Throttle_out]
  [Brake_in] -> TSR System/6
  [Throttle_in] -> TSR System/7
  ISA switch/1 -> TSR System/8
  [Params] -> Bus Selector/1
  SELF_Demux/10(velocity [m/s]) -> TSR System/1, STOPCondition/1(In1), PathFollower_Preview_1/5(velocity [m/s])
  CameraSensor_1_CM_Demux/1(R) -> TSR System/2, CameraSensor_1_CM_Display/1
  CameraSensor_1_CM_Demux/2(G) -> TSR System/3, CameraSensor_1_CM_Display/2
  CameraSensor_1_CM_Demux/3(B) -> TSR System/4, CameraSensor_1_CM_Display/3
  Col/1 -> sat SteeringColumn_pivot_Mux/1
  sat SteeringColumn_pivot_Mux/1 -> d2r SteeringColumn_pivot_Mux/1(Degrees in)
  d2r SteeringColumn_pivot_Mux/1(Radians out) -> SteeringColumn_pivot_Mux/5(Pitch [rad])
  Compare To Constant/1 -> Data Type Conversion/1
  Unit Delay/1 -> Compare To Constant/1
  [Brake_out] -> Unit Delay/1
  Data Type Conversion/1 -> Brake_light_left_Mux/1(MSCD [Cd]), Brake_light_right_Mux/1(MSCD [Cd])
  [Steer] -> Unit Delay2/1
  Unit Delay2/1 -> Gain1/1
  Gain1/1 -> d2r SteeringWheel_pivot_Mux/1(Degrees in)
  d2r SteeringWheel_pivot_Mux/1(Radians out) -> negate SteeringWheel_pivot_Mux/1
  negate SteeringWheel_pivot_Mux/1 -> SteeringWheel_pivot_Mux/4(Roll [rad])
  [Brake_out] -> Dynamics_Simple/3(Brake)
  [Throttle_out] -> Dynamics_Simple/2(Throttle)
  [V_ms] -> JointGroup_WheelDisplacement_V2R/1(Velocity [m/s])
  [Steer] -> Unit Delay1/1
  Unit Delay1/1 -> Gain2/1
  Gain2/1 -> d2r WheelDisplacement_Mux 1/1(Degrees in)
  d2r WheelDisplacement_Mux 1/1(Radians out) -> WheelDisplacement_Mux/1(Steering Angle Front [rad])
  Dynamics_Simple/1(State) -> [State], STATE_Audi_A8_1_rc/1, [State]
  Dynamics_Simple/3(Perf_Params) -> [Params], [Dynamics2PathFollower]
  PathFollower_Preview_1/3(brake pressure [bar]) -> [Brake_in]
  PathFollower_Preview_1/2(throttle [%]) -> [Throttle_in]
  SELF_Demux/4(rotx [deg]) -> [Rotx]
  SELF_Demux/5(roty [deg]) -> [Roty]
  Dynamics_Simple/2(Vx [m s-1]) -> [V_ms]
  PathFollower_Preview_1/1(delta_steerwheel [deg]) -> [Steer], Dynamics_Simple/1(DeltaSteer_[deg])
  Mux/1 -> PathFollower_Preview_1/2(position x,y,Y [m,m,deg])
  SELF_Demux/1(x [m]) -> Mux/1
  SELF_Demux/2(y [m]) -> Mux/2
  SELF_Demux/6(rotz [deg]) -> Mux/3
  V/1 -> PathFollower_Preview_1/3(Initial Velocity [m/s]), PathFollower_Preview_1/4(Desired Velocity [m/s])
  STATE_Audi_A8_1_rc/1 -> STATE_Audi_A8_1_bus/1
  SELF_Audi_A8_1/1 -> SELF_Demux/1(SELF)
  CameraSensor_1/1 -> CameraSensor_1_CM_Demux/1(In1)
  WheelDisplacement_Mux/1(WheelL0_Audi_A8_1) -> WheelL0_Audi_A8_1/1
  WheelDisplacement_Mux/2(WheelL1_Audi_A8_1) -> WheelL1_Audi_A8_1/1
  WheelDisplacement_Mux/3(WheelR0_Audi_A8_1) -> WheelR0_Audi_A8_1/1
  WheelDisplacement_Mux/4(WheelR1_Audi_A8_1) -> WheelR1_Audi_A8_1/1
  JointGroup_WheelDisplacement_V2R/1(Rotation [rad]) -> WheelDisplacement_Mux/3(Rotation [rad])
  SteeringWheel_pivot_Mux/1(Joint) -> SteeringWheel_pivot_Audi_A8_1/1
  SteeringColumn_pivot_Mux/1(Joint) -> SteeringColumn_pivot_Audi_A8_1/1
  Brake_light_left_Mux/1(Lights) -> Audi_A8_1_Brake_light_left/1
  BrakeLightL_Pos/1 -> Brake_light_left_Mux/2(Position (xyz) [m])
  BrakeLightL_Ori/1 -> Brake_light_left_Mux/3(Orientation (RPY) [deg])
  BrakeLightL_Col/1 -> Brake_light_left_Mux/4(Color [-])
  BrakeLightL_ID/1 -> Brake_light_left_Mux/5(TextureResourceID [-])
  Brake_light_right_Mux/1(Lights) -> Audi_A8_1_Brake_light_right/1
  BrakeLightR_Pos/1 -> Brake_light_right_Mux/2(Position (xyz) [m])
  BrakeLightR_Ori/1 -> Brake_light_right_Mux/3(Orientation (RPY) [deg])
  BrakeLightR_Col/1 -> Brake_light_right_Mux/4(Color [-])
  BrakeLightR_ID/1 -> Brake_light_right_Mux/5(TextureResourceID [-])
  Indicator_front_left_Mux/1(Lights) -> Audi_A8_1_Indicator_front_left/1
  IndicatorFL_mscd/1 -> Indicator_front_left_Mux/1(MSCD [Cd])
  IndicatorFL_Pos/1 -> Indicator_front_left_Mux/2(Position (xyz) [m])
  IndicatorFL_Ori/1 -> Indicator_front_left_Mux/3(Orientation (RPY) [deg])
  IndicatorFL_Col/1 -> Indicator_front_left_Mux/4(Color [-])
  IndicatorFL_ID/1 -> Indicator_front_left_Mux/5(TextureResourceID [-])
  Indicator_rear_left_Mux/1(Lights) -> Audi_A8_1_Indicator_rear_left/1
  IndicatorRL_mscd/1 -> Indicator_rear_left_Mux/1(MSCD [Cd])
  IndicatorRL_Pos/1 -> Indicator_rear_left_Mux/2(Position (xyz) [m])
  IndicatorRL_Ori/1 -> Indicator_rear_left_Mux/3(Orientation (RPY) [deg])
  IndicatorRL_Col/1 -> Indicator_rear_left_Mux/4(Color [-])
  IndicatorRL_ID/1 -> Indicator_rear_left_Mux/5(TextureResourceID [-])
  Indicator_front_right_Mux/1(Lights) -> Audi_A8_1_Indicator_front_right/1
  IndicatorFR_mscd/1 -> Indicator_front_right_Mux/1(MSCD [Cd])
  IndicatorFR_Pos/1 -> Indicator_front_right_Mux/2(Position (xyz) [m])
  IndicatorFR_Ori/1 -> Indicator_front_right_Mux/3(Orientation (RPY) [deg])
  IndicatorFR_Col/1 -> Indicator_front_right_Mux/4(Color [-])
  IndicatorFR_ID/1 -> Indicator_front_right_Mux/5(TextureResourceID [-])
  Indicator_rear_right_Mux/1(Lights) -> Audi_A8_1_Indicator_rear_right/1
  IndicatorRR_mscd/1 -> Indicator_rear_right_Mux/1(MSCD [Cd])
  IndicatorRR_Pos/1 -> Indicator_rear_right_Mux/2(Position (xyz) [m])
  IndicatorRR_Ori/1 -> Indicator_rear_right_Mux/3(Orientation (RPY) [deg])
  IndicatorRR_Col/1 -> Indicator_rear_right_Mux/4(Color [-])
  IndicatorRR_ID/1 -> Indicator_rear_right_Mux/5(TextureResourceID [-])
  susp_front/1 -> PathFollower_Preview_1/9(CorneringStiffness_Tyres_Front [N/rad])
  susp_rear/1 -> PathFollower_Preview_1/10(CorneringStiffness_Tyres_Rear [N/rad])
  steering_ratio/1 -> PathFollower_Preview_1/11(steering_ratio[-])
  [State] -> State2PathFollowerCnv/1(State BUS)
  State2PathFollowerCnv/1(Yaw rate [deg/s]) -> PathFollower_Preview_1/8(Yaw rate [deg/s])
  PathFollower_Preview_1/4(v0 [m/s]) -> Dynamics_Simple/4(Initial_Vx_[ms-1])
  PathFollower_Preview_1/5(Auto_GearShift) -> Dynamics_Simple/6(Auto_GearShift)
  FromDynamics2PathFollowerBusSelector/1 -> PathFollower_Preview_1/6(vx [m/s])  "<vx_[ms-1]>"
  FromDynamics2PathFollowerBusSelector/2 -> PathFollower_Preview_1/7(vy [m/s])  "<vy_[ms-1]>"
  [Dynamics2PathFollower] -> FromDynamics2PathFollowerBusSelector/1
  Ground_1/1 -> Dynamics_Simple/5(AutoManual_OnOff)
  Ground_2/1 -> Dynamics_Simple/7(Manual_GearShift)
  Ground_3/1 -> PathFollower_Preview_1/1(ActorOffset_Left(+) / Right(-) [m])
  PathFollower_Preview_1/6(Actor/Traj_distance [m]) -> Terminator_1/1
  PathFollower_Preview_1/7(Actor/Traj_angle [deg]) -> Terminator_2/1
  SELF_Demux/3(z [m]) -> Terminator_3/1
  SELF_Demux/7(GPS lat [deg]) -> Terminator_4/1
  SELF_Demux/8(GPS long [deg]) -> Terminator_5/1
  SELF_Demux/9(GPS alt [m]) -> Terminator_6/1
  SELF_Demux/11(heading [deg]) -> Terminator_7/1
  SELF_Demux/12(yaw rate [deg/s]) -> Terminator_8/1
  State2PathFollowerCnv/2(velocity [m/s]) -> Terminator_9/1
  State2PathFollowerCnv/3(position x,y,Y [m,m,deg]) -> Terminator_10/1
  Ground_4/1 -> SteeringColumn_pivot_Mux/1(X [m])
  Ground_5/1 -> SteeringColumn_pivot_Mux/2(Y [m])
  Ground_6/1 -> SteeringColumn_pivot_Mux/3(Z [m])
  Ground_7/1 -> SteeringColumn_pivot_Mux/4(Roll [rad])
  Ground_8/1 -> SteeringColumn_pivot_Mux/6(Yaw [rad])
  Ground_9/1 -> SteeringWheel_pivot_Mux/1(X [m])
  Ground_10/1 -> SteeringWheel_pivot_Mux/2(Y [m])
  Ground_11/1 -> SteeringWheel_pivot_Mux/3(Z [m])
  Ground_12/1 -> SteeringWheel_pivot_Mux/5(Pitch [rad])
  Ground_13/1 -> SteeringWheel_pivot_Mux/6(Yaw [rad])
  TSR System/3 -> Terminator_11/1
  Ground_14/1 -> WheelDisplacement_Mux/2(Steering Angle Rear [rad])

== system TSR_EuroNCAP_MSA_ISA_cs/Audi_A8_1_Brake_light_left ==
  Audi_A8_1_Brake_light_left : Inport  Tag=inport/BrakeLightL  OutDataTypeStr=Bus: PRESCAN_VISULIGHTACTUATOR_DATA  SampleTime=1/100  BusOutputAsStruct=on
  Actuator : S-Function  FunctionName=sfun_VisuLightActuator  Parameters=mbxruntime.parameters.convert(UniqueID), mbxruntime.parameters.convert(LightName), mbxruntime.parameters.convert(PivotName), mbxruntime.parameters.convert(TextureResources), mbxruntime.parameters.convert(ColorsObjectName), mbxruntime.parameters.convert(MeshOnColor), mbxruntime.parameters.convert(MeshOffColor),tabledata, TimeStep  EnableBusSupport=off  mask(PreScan Sink Block: VisuActiveLight){UniqueID=253, LightName=Audi_A8_1.LightActuator_0_BrakeLightRL_ActiveLight, PivotName=Audi_A8_1.BrakeLightL_pivot, TextureResources={ '9' 'LightMap\GeneralLight.png'}, ColorsObjectName=Audi_A8_1.BrakeLightRL, MeshOnColor=[255    0    0  255  255    0    0  255  102  102  102  255  510    0    0  255], MeshOffColor=[255    0    0  255  255    0    0  255  102  102  102  255    0    0    0  255], TimeStep=1/100}
      mask prompts: UniqueID "Parent Unique Identifier"; LightName "Light"; PivotName "Pivot"; TextureResources "Texture Resources"; ColorsObjectName "Light Fixture Color Object"; MeshOnColor "Light Fixture On Color"; MeshOffColor "Light Fixture Off Color"; TimeStep "Simulink time step"
      mask help:
      | The VisuActiveLight block provides a way for detailed animation of Light Sources, such as the indicator, brake, fog and main lights of a vehicle, or a light post.
      |
      | For more information, please click Help.
      mask init:
      | [tabledata] = mbxruntime.parameters.table(UniqueID,LightName,PivotName,TextureResources,ColorsObjectName,MeshOnColor,MeshOffColor);
      mask Help: eval('openHelp(209)')
      mask Display: image(imread('HeadLight.png'))
  wires:
  Audi_A8_1_Brake_light_left/1 -> Actuator/1

== system TSR_EuroNCAP_MSA_ISA_cs/Audi_A8_1_Brake_light_right ==
  Audi_A8_1_Brake_light_right : Inport  Tag=inport/BrakeLightR  OutDataTypeStr=Bus: PRESCAN_VISULIGHTACTUATOR_DATA  SampleTime=1/100  BusOutputAsStruct=on
  Actuator : S-Function  FunctionName=sfun_VisuLightActuator  Parameters=mbxruntime.parameters.convert(UniqueID), mbxruntime.parameters.convert(LightName), mbxruntime.parameters.convert(PivotName), mbxruntime.parameters.convert(TextureResources), mbxruntime.parameters.convert(ColorsObjectName), mbxruntime.parameters.convert(MeshOnColor), mbxruntime.parameters.convert(MeshOffColor),tabledata, TimeStep  EnableBusSupport=off  mask(PreScan Sink Block: VisuActiveLight){UniqueID=253, LightName=Audi_A8_1.LightActuator_1_BrakeLightRR_ActiveLight, PivotName=Audi_A8_1.BrakeLightR_pivot, TextureResources={ '9' 'LightMap\GeneralLight.png'}, ColorsObjectName=Audi_A8_1.BrakeLightRR, MeshOnColor=[255    0    0  255  255    0    0  255  102  102  102  255  510    0    0  255], MeshOffColor=[255    0    0  255  255    0    0  255  102  102  102  255    0    0    0  255], TimeStep=1/100}
      mask prompts: UniqueID "Parent Unique Identifier"; LightName "Light"; PivotName "Pivot"; TextureResources "Texture Resources"; ColorsObjectName "Light Fixture Color Object"; MeshOnColor "Light Fixture On Color"; MeshOffColor "Light Fixture Off Color"; TimeStep "Simulink time step"
      mask help:
      | The VisuActiveLight block provides a way for detailed animation of Light Sources, such as the indicator, brake, fog and main lights of a vehicle, or a light post.
      |
      | For more information, please click Help.
      mask init:
      | [tabledata] = mbxruntime.parameters.table(UniqueID,LightName,PivotName,TextureResources,ColorsObjectName,MeshOnColor,MeshOffColor);
      mask Help: eval('openHelp(209)')
      mask Display: image(imread('HeadLight.png'))
  wires:
  Audi_A8_1_Brake_light_right/1 -> Actuator/1
